simulink model "MPC_Kalman"  (R2024b)
settings: Solver=VariableStepAuto  StartTime=0.0  StopTime=50  RelTol=1e-3
values from neighbouring files (symbols this model uses):
  B_noise = [Bz ones(size(Bz,1),1)]    [main.m]
  C_state = eye(12)    [main.m]
  D_noise = [D_state zeros(size(D_state,1),1)]    [main.m]
  NK = 0    [main.m]
  Q_LQ = q * eye(12)    [main.m]
  R_LQ = r    (= 1e-05)    [main.m]
  RK = r    (= 1e-05)    [main.m]
  S = zeros(n)    [main.m]
  Ts = 0.1    [main.m]    (also in point7.m)
  Ubar_z = inv(dcgain(Gz))*Ybar    [main.m]
  umax = +15    (= 15)    [main.m]
  umin = -15    [main.m]
  x0 = [3,0,3,0,3,0,3,0,3,0,3,0]    [main.m]
  x0K = 1.5*x0    [main.m]
  Xbar_z = (eye(12) - Az) \ (Bz * Ubar_z)    [main.m]
  xmax = [ 10;  Inf;  10;  Inf;  10;  Inf;  10;  Inf;  10;  Inf;  10;  Inf]    [main.m]
  xmin = [-10; -Inf; -10; -Inf; -10; -Inf; -10; -Inf; -10; -Inf; -10; -Inf]    [main.m]
undefined symbols (not defined in the file or in its folder): Az, Bz, Cz, Discrete, Dz, mympc_project_constraints, Time
libraries: simulink x2, ctrlSharedLib x1
settings Model: Creator=faiol  LastModifiedBy=faiol

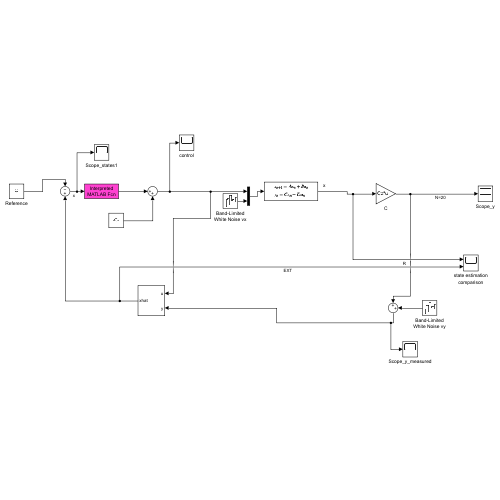
[thumbnail: Simulink's stored preview of the top-level diagram]
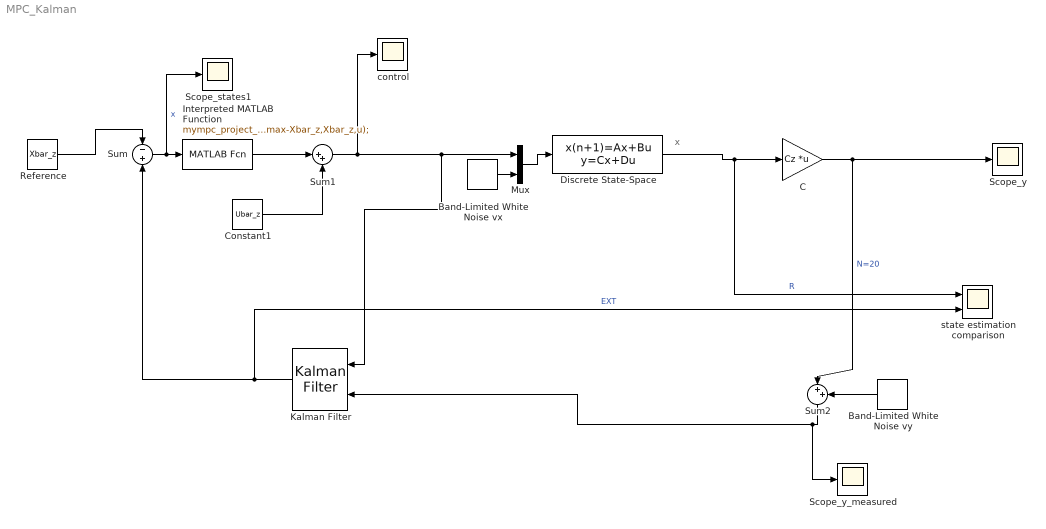
== system MPC_Kalman ==
  note: x
  Band-Limited White Noise vx : simulink/Sources/Band-Limited White Noise  Cov=power_vx  Ts=Ts  seed=[23341]
  Band-Limited White Noise vy : simulink/Sources/Band-Limited White Noise  Cov=power_vy  Ts=Ts  seed=[23341]
  C : Gain  Gain=Cz  Multiplication=Matrix(K*u)
  Constant1 : Constant  Value=Ubar_z  SampleTime=Ts
  Discrete State-Space : DiscreteStateSpace  A=Az  B=B_noise  C=C_state  D=D_noise  InitialCondition=x0  SampleTime=Ts
  Interpreted MATLAB Function : MATLABFcn  MATLABFcn=mympc_project_constraints(Az,Bz,Q_LQ,R_LQ,S,20,umin-Ubar_z,umax-Ubar_z,Ubar_z,xmin-Xbar_z,xmax-Xbar_z,Xbar_z,u);  OutputDimensions=1
  Kalman Filter : ctrlSharedLib/Kalman Filter  TimeDomain=Discrete-Time  UseCurrentEstimator=on  ModelSource=Individual A, B, C, D matrices  ModelSourceVariable=ss(0.95,1,1,0,1)  A=Az  B=Bz  C=Cz  D=Dz  NumberOfStates=1  NumberOfInputs=1  NumberOfOutputs=1  InitialEstimateSource=Dialog  X0=x0K  P0=10  UseK=off  UseGH=off  NumberOfProcessNoiseInputs=1  G=1  TimeInvariantG=on  H=0  TimeInvariantH=on  Q=QK  TimeInvariantQ=on  R=RK  TimeInvariantR=on  N=NK  TimeInvariantN=on  AddInputPort=on  AddEnablePort=off  OutputEstimatedY=off  OutputP=off  Ts=Ts
  Mux : Mux  Inputs=2
  Reference : Constant  Value=Xbar_z  SampleTime=Ts
  Scope_states1 : Scope
  Scope_y : Scope
  Scope_y_measured : Scope
  Sum : Sum  Inputs=-+
  Sum1 : Sum  Inputs=|++
  Sum2 : Sum  Inputs=|++
  control : Scope
  "state estimation comparison " : Scope  NumInputPorts=2
  wires:
  Sum1/1 -> Mux/1, Kalman Filter/1, control/1
  Sum/1 -> Scope_states1/1, Interpreted MATLAB Function/1  "x"
  C/1 -> Scope_y/1, Sum2/1  "N=20"
  Discrete State-Space/1 -> "state estimation comparison "/1, C/1  "R"
  Interpreted MATLAB Function/1 -> Sum1/1
  Band-Limited White Noise vx/1 -> Mux/2
  Kalman Filter/1 -> "state estimation comparison "/2, Sum/2  "EXT"
  Band-Limited White Noise vy/1 -> Sum2/2
  Sum2/1 -> Scope_y_measured/1, Kalman Filter/2
  Mux/1 -> Discrete State-Space/1
  Constant1/1 -> Sum1/2
  Reference/1 -> Sum/1
